simulink model "base_simulink"  (R2021b)
settings: Solver=FixedStepAuto  StartTime=0.0  StopTime=6  FixedStep=0.00005  RelTol=1e-3
undefined symbols (not defined in the file): sigbuilder_block, X, Y, Z
libraries: sm_lib x64, nesl_utility x18, slpidlib x8
(part 3 of 3)

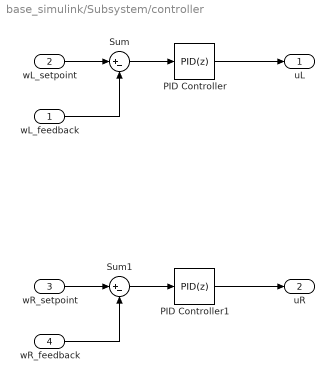
== system base_simulink/Subsystem/controller ==
  wL_feedback : Inport
  wL_setpoint : Inport  Port=2
  wR_setpoint : Inport  Port=3
  wR_feedback : Inport  Port=4
  PID Controller : slpidlib/PID Controller  Controller=PID  Form=Parallel  TimeDomain=Discrete-time  UseExternalTs=off  SampleTime=0.001  IntegratorMethod=Forward Euler  FilterMethod=Forward Euler  ControllerParametersSource=internal  P=1.5  I=0.6  D=1  UseFilter=on  N=100  TunerSelectOption=Transfer Function Based (PID Tuner App)  InitialConditionSource=internal  InitialConditionForIntegrator=0  InitialConditionForFilter=0  DifferentiatorICPrevScaledInput=0  ExternalReset=none  TrackingMode=off  Kt=1  LimitOutput=off  SatLimitsSource=internal  UpperSaturationLimit=inf  LowerSaturationLimit=-inf  LinearizeAsGain=on  AntiWindupMode=none  Kb=1  POutMin=[]  POutMax=[]  IOutMin=[]  IOutMax=[]  DOutMin=[]  DOutMax=[]  NOutMin=[]  NOutMax=[]  SumOutMin=[]  SumOutMax=[]  SaturationOutMin=[]  SaturationOutMax=[]  PParamMin=[]  PParamMax=[]  IParamMin=[]  IParamMax=[]  DParamMin=[]  DParamMax=[]  NParamMin=[]  NParamMax=[]  KbParamMin=[]  KbParamMax=[]  KtParamMin=[]  KtParamMax=[]  KbOutMin=[]  KbOutMax=[]  KtOutMin=[]  KtOutMax=[]  IntegratorOutMin=[]  IntegratorOutMax=[]  FilterOutMin=[]  FilterOutMax=[]  SumI1OutMin=[]  SumI1OutMax=[]  SumI2OutMin=[]  SumI2OutMax=[]  SumI3OutMin=[]  SumI3OutMax=[]  SumI4OutMin=[]  SumI4OutMax=[]  SumDOutMin=[]  SumDOutMax=[]  DifferentiatorOutMin=[]  DifferentiatorOutMax=[]  FilterDiffOutCoefMin=[]  FilterDiffOutCoefMax=[]  ReciprocalOutMin=[]  ReciprocalOutMax=[]  SumDenOutMin=[]  SumDenOutMax=[]  SumNumOutMin=[]  SumNumOutMax=[]  DivideOutMin=[]  DivideOutMax=[]  UdiffTsProdOutMin=[]  UdiffTsProdOutMax=[]  NTsProdOutMin=[]  NTsProdOutMax=[]  UintegralTsProdOutMin=[]  UintegralTsProdOutMax=[]  UngainTsProdOutMin=[]  UngainTsProdOutMax=[]  IntegratorContinuousStateAttributes=''  IntegratorStateMustResolveToSignalObject=off  IntegratorRTWStateStorageClass=Auto  FilterContinuousStateAttributes=''  FilterStateMustResolveToSignalObject=off  FilterRTWStateStorageClass=Auto  ParallelPVariant=InternalParameters  IdealPVariant=Disabled  IVariant=InternalParameters  DVariant=InternalParameters  IntegratorVariant=Discrete  SatVariant=Disabled  AWVariant=Passthrough  PCopyVariant=Disabled  TRVariant=Disabled  FdbkBlocksVariant=Forward  IdealPFdbkVariant=Disabled  SatFdbkVariant=Disabled  DerivativeFilterVariant=ForwardEulerFilter  NVariant=InternalParameters  NCopyVariant=Disabled  FilterICVariant=InternalICsFilter  IntegratorICVariant=InternalICs  ExternalResetVariant=Disabled  TRSumVariant=Passthrough  SumFdbkVariant=Disabled  SumVariant=Sum_PID  TsampFilterVariant=InternalTs  TsampNgainVariant=Passthrough  TsampIntegralVariant=Passthrough  ExternalSaturationOutDataTypeStr=Inherit: Same as second input
  PID Controller1 : slpidlib/PID Controller  Controller=PID  Form=Parallel  TimeDomain=Discrete-time  UseExternalTs=off  SampleTime=0.001  IntegratorMethod=Forward Euler  FilterMethod=Forward Euler  ControllerParametersSource=internal  P=1.5  I=0.6  D=1  UseFilter=on  N=100  TunerSelectOption=Transfer Function Based (PID Tuner App)  InitialConditionSource=internal  InitialConditionForIntegrator=0  InitialConditionForFilter=0  DifferentiatorICPrevScaledInput=0  ExternalReset=none  TrackingMode=off  Kt=1  LimitOutput=off  SatLimitsSource=internal  UpperSaturationLimit=inf  LowerSaturationLimit=-inf  LinearizeAsGain=on  AntiWindupMode=none  Kb=1  POutMin=[]  POutMax=[]  IOutMin=[]  IOutMax=[]  DOutMin=[]  DOutMax=[]  NOutMin=[]  NOutMax=[]  SumOutMin=[]  SumOutMax=[]  SaturationOutMin=[]  SaturationOutMax=[]  PParamMin=[]  PParamMax=[]  IParamMin=[]  IParamMax=[]  DParamMin=[]  DParamMax=[]  NParamMin=[]  NParamMax=[]  KbParamMin=[]  KbParamMax=[]  KtParamMin=[]  KtParamMax=[]  KbOutMin=[]  KbOutMax=[]  KtOutMin=[]  KtOutMax=[]  IntegratorOutMin=[]  IntegratorOutMax=[]  FilterOutMin=[]  FilterOutMax=[]  SumI1OutMin=[]  SumI1OutMax=[]  SumI2OutMin=[]  SumI2OutMax=[]  SumI3OutMin=[]  SumI3OutMax=[]  SumI4OutMin=[]  SumI4OutMax=[]  SumDOutMin=[]  SumDOutMax=[]  DifferentiatorOutMin=[]  DifferentiatorOutMax=[]  FilterDiffOutCoefMin=[]  FilterDiffOutCoefMax=[]  ReciprocalOutMin=[]  ReciprocalOutMax=[]  SumDenOutMin=[]  SumDenOutMax=[]  SumNumOutMin=[]  SumNumOutMax=[]  DivideOutMin=[]  DivideOutMax=[]  UdiffTsProdOutMin=[]  UdiffTsProdOutMax=[]  NTsProdOutMin=[]  NTsProdOutMax=[]  UintegralTsProdOutMin=[]  UintegralTsProdOutMax=[]  UngainTsProdOutMin=[]  UngainTsProdOutMax=[]  IntegratorContinuousStateAttributes=''  IntegratorStateMustResolveToSignalObject=off  IntegratorRTWStateStorageClass=Auto  FilterContinuousStateAttributes=''  FilterStateMustResolveToSignalObject=off  FilterRTWStateStorageClass=Auto  ParallelPVariant=InternalParameters  IdealPVariant=Disabled  IVariant=InternalParameters  DVariant=InternalParameters  IntegratorVariant=Discrete  SatVariant=Disabled  AWVariant=Passthrough  PCopyVariant=Disabled  TRVariant=Disabled  FdbkBlocksVariant=Forward  IdealPFdbkVariant=Disabled  SatFdbkVariant=Disabled  DerivativeFilterVariant=ForwardEulerFilter  NVariant=InternalParameters  NCopyVariant=Disabled  FilterICVariant=InternalICsFilter  IntegratorICVariant=InternalICs  ExternalResetVariant=Disabled  TRSumVariant=Passthrough  SumFdbkVariant=Disabled  SumVariant=Sum_PID  TsampFilterVariant=InternalTs  TsampNgainVariant=Passthrough  TsampIntegralVariant=Passthrough  ExternalSaturationOutDataTypeStr=Inherit: Same as second input
  Sum : Sum  Inputs=|+-
  Sum1 : Sum  Inputs=|+-
  uL : Outport
  uR : Outport  Port=2
  wires:
  PID Controller/1 -> uL/1
  Sum/1 -> PID Controller/1
  wL_feedback/1 -> Sum/2
  wL_setpoint/1 -> Sum/1
  wR_setpoint/1 -> Sum1/1
  Sum1/1 -> PID Controller1/1
  wR_feedback/1 -> Sum1/2
  PID Controller1/1 -> uR/1

== system base_simulink/Subsystem/base/External Load ==
  Brick Solid : sm_lib/Body Elements/Brick Solid  GraphicAmbientColor=[0.15 0.15 0.15 1.0]  BasedOnType=Mass  BrickDimensions=[50 50 50]  BrickDimensionUnits=mm  CenterOfMass=[0 0 0]  CenterOfMassUnits=m  GraphicDiffuseColor=[0.5 0.5 0.5]  Density=1000  DensityUnits=kg/m^3  DoExposeReferenceFrame=on  GraphicEmissiveColor=[0.0 0.0 0.0 1.0]  ExportEntireGeometry=off  SerializedFrames=<Frames/>  MarkerShape=Sphere  MarkerSize=10  GraphicType=FromGeometry  InertiaType=CalculateFromGeometry  Mass=50  MassUnits=g  MomentsOfInertia=[1 1 1]  MomentsOfInertiaUnits=kg*m^2  GraphicOpacity=1.0  ProductsOfInertia=[0 0 0]  ProductsOfInertiaUnits=kg*m^2  GraphicShininess=75  GraphicSpecularColor=[0.5 0.5 0.5 1.0]  GraphicVisPropType=SimpleVisualProperties
  Rigid Transform14 : sm_lib/Frames and Transforms/Rigid Transform  TranslationMethod=StandardAxis  TranslationStandardOffset=40.25  TranslationLengthUnit=mm  TranslationStandardAxis=+Z  TranslationCartesianOffset=[0 0 0]  TranslationROffset=0  TranslationROffsetUnits=m  TranslationZOffset=0  TranslationZOffsetUnits=m  TranslationThetaOffset=0  TranslationThetaOffsetUnits=deg  RotationMethod=None  RotationAngleUnits=deg  RotationStandardAxis=+Z  RotationAngle=0.0  RotationArbitraryAxis=[0 0 1]  FollAlignAxisA=+X  BaseAlignAxisA=+Y  FollAlignAxisB=+Y  BaseAlignAxisB=+Z  RotationSequenceAxes=FollowerAxes  RotationSequence=XYX  RotationSequenceAngles=[0 0 0]  RotationSequenceAnglesUnits=deg  RotationMatrix=[1 0 0; 0 1 0; 0 0 1]
  Conn1 : PMIOPort  Side=Left
  connections:
  Rigid Transform14/RConn1 -- Brick Solid/RConn1
  Rigid Transform14/LConn1 -- Conn1/RConn1

== matlab function base_simulink/Subsystem/Kalman filter L/Kalman filter ==
  data: theta_k input; X1 output; X1 input; X2 input; P11 input; P12 input; P21 input; P22 input; X2 output; PP11 output; PP12 output; PP21 output; PP22 output; dP output
function [X1,X2,PP11,PP12,PP21,PP22,dP] = KalmanFilterFNC(theta_k,X1,X2,P11,P12,P21,P22)
%syms delta_t theta_k omega_k V_k Q x_k1 xp_hat_k x_hat_k P_hat_k yp_k R x11 x21 p11 p12 p21 p22 dt
dt = 0.0001;
omega_k = 0;
delta_t = dt;
A = [1 delta_t;0 1];
G = [delta_t*delta_t/2;delta_t];
C = [1 0];
Q = 6.800;
R = 0.01;
x_k = [theta_k;0]
%x_k = A*x_k1;
y_k = C*x_k;
x11 = X1;
x21 = X2;
x_hat_k = [x11;x21]
p11 = P11;
p12 = P12;
p21 = P21;
p22 = P22;
P_hat_k = [p11 p12;p21 p22];

%pred -------------------------------------

xp_hat_k = A*x_hat_k;
Pp_hat_k = A*P_hat_k*transpose(A) + G*Q*transpose(G);

%upadate

yp_k = C*xp_hat_k;
y_re_k = y_k - yp_k;
S_k = C*Pp_hat_k*transpose(C) + R;
K_k = Pp_hat_k*transpose(C)/(S_k);
x_hat_k1 = xp_hat_k+K_k*y_re_k;
P_hat_k1 = ([1 0;0 1]-(K_k*C))*Pp_hat_k;

%X1 = x_hat_k1(1);
%X2 = x_hat_k1(2);
%PP11 = P_hat_k1(1,1);
%PP12 = P_hat_k1(1,2);
%PP21 = P_hat_k1(2,1);
%PP22 =P_hat_k1(2,2);
X1 = X1 + X2*dt - ((X1 - theta_k + X2*dt)*(P11 + P21*dt + (Q*dt^4)/4 + dt*(P12 + P22*dt)))/(P11 + R + P21*dt + (Q*(dt^4))/4 + dt*(P12 + P22*dt));
X2 = X2 - (((Q*(dt^3))/2 + P22*dt + P21)*(X1 - theta_k + X2*dt))/(P11 + R + P21*dt + (Q*(dt^4))/4 + dt*(P12 + P22*dt));
PP11 = -((P11 + P21*dt + (Q*(dt^4))/4 + dt*(P12 + P22*dt))/(P11 + R + P21*dt + (Q*(dt^4))/4 + dt*(P12 + P22*dt)) - 1)*(P11 + P21*dt + (Q*(dt^4))/4 + dt*(P12 + P22*dt));
PP12 = -((P11 + P21*dt + (Q*(dt^4))/4 + dt*(P12 + P22*dt))/(P11 + R + P21*dt + (Q*(dt^4))/4 + dt*(P12 + P22*dt)) - 1)*((Q*(dt^3))/2 + P22*dt + P12);
PP21 = P21 + P22*dt + (Q*(dt^3))/2 - (((Q*(dt^3))/2 + P22*dt + P21)*(P11 + P21*dt + (Q*(dt^4))/4 + dt*(P12 + P22*dt)))/(P11 + R + P21*dt + (Q*(dt^4))/4 + dt*(P12 + P22*dt));
PP22 = P22 + Q*(dt^2) - (((Q*(dt^3))/2 + P22*dt + P12)*((Q*(dt^3))/2 + P22*dt + P21))/(P11 + R + P21*dt + (Q*(dt^4))/4 + dt*(P12 + P22*dt));
dP = det([PP11 PP12;PP21 PP22])

== matlab function base_simulink/Subsystem/IK ==
  data: v input; wL output; w input; R input; L input; wR output
function [wL,wR] = IK(v,w,R,L)
wL = (1/R)*(v-(w*L)/2);
wR = (1/R)*(v+(w*L)/2);

== matlab function base_simulink/Subsystem/Kalman filter R/Kalman filter ==
  data: theta_k input; X1 output; X1 input; X2 input; P11 input; P12 input; P21 input; P22 input; X2 output; PP11 output; PP12 output; PP21 output; PP22 output; dP output
function [X1,X2,PP11,PP12,PP21,PP22,dP] = KalmanFilterFNC(theta_k,X1,X2,P11,P12,P21,P22)
%syms delta_t theta_k omega_k V_k Q x_k1 xp_hat_k x_hat_k P_hat_k yp_k R x11 x21 p11 p12 p21 p22 dt
dt = 0.0001;
omega_k = 0;
delta_t = dt;
A = [1 delta_t;0 1];
G = [delta_t*delta_t/2;delta_t];
C = [1 0];
Q = 6.800;
R = 0.01;
x_k = [theta_k;0]
%x_k = A*x_k1;
y_k = C*x_k;
x11 = X1;
x21 = X2;
x_hat_k = [x11;x21]
p11 = P11;
p12 = P12;
p21 = P21;
p22 = P22;
P_hat_k = [p11 p12;p21 p22];

%pred -------------------------------------

xp_hat_k = A*x_hat_k;
Pp_hat_k = A*P_hat_k*transpose(A) + G*Q*transpose(G);

%upadate

yp_k = C*xp_hat_k;
y_re_k = y_k - yp_k;
S_k = C*Pp_hat_k*transpose(C) + R;
K_k = Pp_hat_k*transpose(C)/(S_k);
x_hat_k1 = xp_hat_k+K_k*y_re_k;
P_hat_k1 = ([1 0;0 1]-(K_k*C))*Pp_hat_k;

%X1 = x_hat_k1(1);
%X2 = x_hat_k1(2);
%PP11 = P_hat_k1(1,1);
%PP12 = P_hat_k1(1,2);
%PP21 = P_hat_k1(2,1);
%PP22 =P_hat_k1(2,2);
X1 = X1 + X2*dt - ((X1 - theta_k + X2*dt)*(P11 + P21*dt + (Q*dt^4)/4 + dt*(P12 + P22*dt)))/(P11 + R + P21*dt + (Q*(dt^4))/4 + dt*(P12 + P22*dt));
X2 = X2 - (((Q*(dt^3))/2 + P22*dt + P21)*(X1 - theta_k + X2*dt))/(P11 + R + P21*dt + (Q*(dt^4))/4 + dt*(P12 + P22*dt));
PP11 = -((P11 + P21*dt + (Q*(dt^4))/4 + dt*(P12 + P22*dt))/(P11 + R + P21*dt + (Q*(dt^4))/4 + dt*(P12 + P22*dt)) - 1)*(P11 + P21*dt + (Q*(dt^4))/4 + dt*(P12 + P22*dt));
PP12 = -((P11 + P21*dt + (Q*(dt^4))/4 + dt*(P12 + P22*dt))/(P11 + R + P21*dt + (Q*(dt^4))/4 + dt*(P12 + P22*dt)) - 1)*((Q*(dt^3))/2 + P22*dt + P12);
PP21 = P21 + P22*dt + (Q*(dt^3))/2 - (((Q*(dt^3))/2 + P22*dt + P21)*(P11 + P21*dt + (Q*(dt^4))/4 + dt*(P12 + P22*dt)))/(P11 + R + P21*dt + (Q*(dt^4))/4 + dt*(P12 + P22*dt));
PP22 = P22 + Q*(dt^2) - (((Q*(dt^3))/2 + P22*dt + P12)*((Q*(dt^3))/2 + P22*dt + P21))/(P11 + R + P21*dt + (Q*(dt^4))/4 + dt*(P12 + P22*dt));
dP = det([PP11 PP12;PP21 PP22])

== matlab function base_simulink/Subsystem/MATLAB Function ==
  data: wL input; v output; wR input; R input; L input; w output
function [v,w] = FK(wL,wR,R,L)
v = (R/2)*(wL+wR);
w = (R/L)*(wR-wL);
